simulink model "four_phase_iek_dynamic_load_refslew"  (R2024b)
settings: Solver=VariableStepAuto  StartTime=0.0  StopTime=2e-3  MaxStep=max_step_cont  RelTol=1e-3
undefined symbols (not defined in the file): Cout, DCR_L1, DCR_L2, DCR_L3, DCR_L4, ESR_C, IL_adc_counts_per_A, IL_pk_limit_adc_neg, IL_pk_limit_adc_pos, Iload_final, Iload_initial, Iqcot_enable, Kiqcot, L, Lambda1, Lambda2, Lambda3, Lambda4, Ri_area, t_load_step, Tblank, Tdead, Tiqcot_leak, Toff_min, Ton_cmd, Ton_iq_max, Ton_iq_min, Ton_trim1, Ton_trim2, Ton_trim3, Ton_trim4, Tslot, Tss, Varea_bias, Vcot_ramp_amp, Vcot_ramp_enable, Vhys, Vin, Vo_ref
libraries: simulink x29, spsCurrentMeasurementLib x8, spsMosfetLib x8, spsSeriesRLCBranchLib x5, spsVoltageMeasurementLib x5, spsDCVoltageSourceLib x4, spsControlledCurrentSourceLib x1, spsGroundLib x1, spspowerguiLib x1
settings Model: Creator=zengruize  LastModifiedBy=zengruize

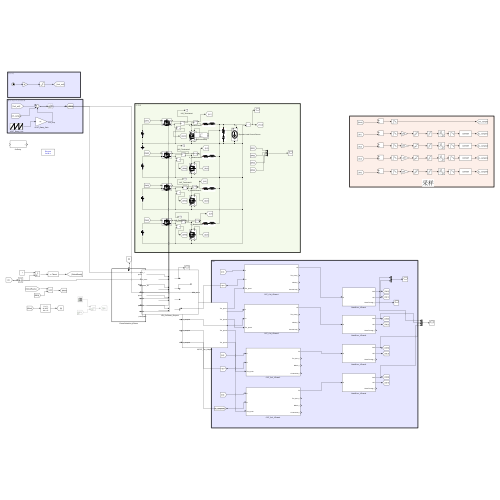
[thumbnail: Simulink's stored preview of the top-level diagram]
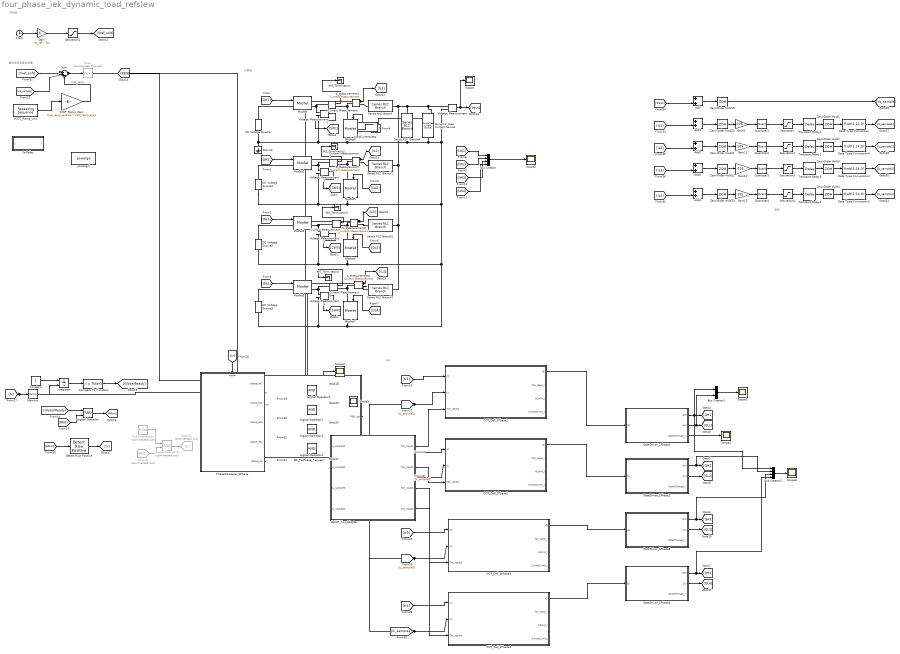
== system four_phase_iek_dynamic_load_refslew ==
  note: cot
  note: 输出电压误差比较器
  note: 功率级
  note: 软启动
  note: 采样
  Add{,1..4} (5 alike) : Sum
  Bus Creator : BusCreator  Inputs=4
  Bus Creator1 : BusCreator  Inputs=2
  Bus Creator2 : BusCreator  Inputs=4
  COT_Cell_1Phase1 : Subsystem
  COT_Cell_1Phase2 : Subsystem
  COT_Cell_1Phase3 : Subsystem
  COT_Cell_1Phase4 : Subsystem
  Clock : Clock
  Compare To Constant : simulink/Logic and Bit Operations/Compare To Constant  relop=>=  const=Tblank  OutDataTypeStr=boolean
  Constant : Constant
  Current Measurement{,1..3} (4 alike) : spsCurrentMeasurementLib/Current Measurement  PhasorSimulation=off  OutputType=Complex  PSBequivalent=0
  DC Voltage Source{,1..3} (4 alike) : spsDCVoltageSourceLib/DC Voltage Source  Amplitude=Vin  Measurements=None
  Data Type Conversion{,2..4} (4 alike) : DataTypeConversion  OutDataTypeStr=fixdt(1,14,0)  SaturateOnIntegerOverflow=off  RndMeth=Floor
  Detect Rise Positive : simulink/Logic and Bit Operations/Detect Rise Positive  vinit=0  OutDataTypeStr=boolean
  Dynamic Load Current Source : spsControlledCurrentSourceLib/Controlled Current Source  Initialize=on  Source_Type=DC  Amplitude=0  Phase=0  Frequency=0  Measurements=None
  From31 : From  Commented=on  GotoTag=REQ
  Gain : Gain  Gain=Vo_ref / Tss
  Gain11 : Gain  Gain=205
  Gain12 : Gain  Gain=-205
  Gain13 : Gain  Gain=205
  Gain9 : Gain  Gain=-205
  GateDriver_1Phase1 : Subsystem
  GateDriver_1Phase2 : Subsystem
  GateDriver_1Phase3 : Subsystem
  GateDriver_1Phase4 : Subsystem
  Goto26 : Goto  Commented=on  GotoTag=tr
  Ground : spsGroundLib/Ground  LConnTagsString=a
  IEK_PerPhase_Request : Subsystem
  IHS_Terminator{1..4} (4 alike) : Terminator
  IL_Measurement{1..4} (4 alike) : spsCurrentMeasurementLib/Current Measurement  PhasorSimulation=off  OutputType=Complex  PSBequivalent=0
  IQCOT_Ton_Adapter : Subsystem
  Integrator : Integrator  ExternalReset=rising
  LoadCurrentStep : Step  Time=t_load_step  Before=Iload_initial  After=Iload_final  SampleTime=0
  Logical Operator{,1..4} (5 alike) : Logic  AllPortsSameDT=off  OutDataTypeStr=boolean
  Logical Operator5 : Logic  Commented=on  AllPortsSameDT=off  OutDataTypeStr=boolean
  Memory : Memory
  Mosfet{,1..3} (4 alike) : spsMosfetLib/Mosfet  Ron=Ron_HS  Lon=0  Rd=Rd_body  Vfd=Vfd_body  IC=0  Rs=Rs_snubber  Cs=Cs_snubber  Measurements=on
  Mosfet{4..7} (4 alike) : spsMosfetLib/Mosfet  Ron=Ron_LS  Lon=0  Rd=Rd_body  Vfd=Vfd_body  IC=0  Rs=Rs_snubber  Cs=Cs_snubber  Measurements=on
  OnDelay : Subsystem
  PhaseScheduler_4Phase : Subsystem  TreatAsAtomicUnit=on
  Pulse Generator : DiscretePulseGenerator  Commented=on  PulseType=Time based  Period=Tblank  PulseWidth=5
  Quantizer{1..4} (4 alike) : Quantizer  QuantizationInterval=1
  Relay : Relay  Commented=through  OnSwitchValue=Vhys/2  OffSwitchValue=-Vhys/2
  Saturation{,1,3..4} (4 alike) : Saturate  UpperLimit=8191  LowerLimit=-8191
  Saturation2 : Saturate  UpperLimit=Vo_ref  LowerLimit=0
  Scope{,1..6} (7 alike) : Scope
  Series RLC Branch : spsSeriesRLCBranchLib/Series RLC Branch  LConnTagsString=__new0  RConnTagsString=__new0  BranchType=RL  Resistance=DCR_L1  Inductance=L  SetiL0=off  InitialCurrent=0  Capacitance=1e-6  Setx0=off  InitialVoltage=0  Measurements=None
  Series RLC Branch1 : spsSeriesRLCBranchLib/Series RLC Branch  LConnTagsString=__new0  RConnTagsString=__new0  BranchType=RL  Resistance=DCR_L2  Inductance=L  SetiL0=off  InitialCurrent=0  Capacitance=1e-6  Setx0=off  InitialVoltage=0  Measurements=None
  Series RLC Branch2 : spsSeriesRLCBranchLib/Series RLC Branch  LConnTagsString=__new0  RConnTagsString=__new0  BranchType=RL  Resistance=DCR_L3  Inductance=L  SetiL0=off  InitialCurrent=0  Capacitance=1e-6  Setx0=off  InitialVoltage=0  Measurements=None
  Series RLC Branch3 : spsSeriesRLCBranchLib/Series RLC Branch  LConnTagsString=__new0  RConnTagsString=__new0  BranchType=RL  Resistance=DCR_L4  Inductance=L  SetiL0=off  InitialCurrent=0  Capacitance=1e-6  Setx0=off  InitialVoltage=0  Measurements=None
  Series RLC Branch4 : spsSeriesRLCBranchLib/Series RLC Branch  LConnTagsString=__new0  RConnTagsString=__new0  BranchType=RC  Resistance=ESR_C  Inductance=1e-3  SetiL0=off  InitialCurrent=0  Capacitance=Cout  Setx0=on  InitialVoltage=Vo_ref  Measurements=None
  Sum : Sum  Inputs=|+--
  Transport Delay{1..4} (4 alike) : TransportDelay  DelayTime=5/25000000
  VCOT_Ramp_Gain : Gain  Gain=Vcot_ramp_enable * Vcot_ramp_amp
  VCOT_Ramp_Unit : simulink/Sources/Repeating Sequence  rep_seq_t=[0 Tslot]  rep_seq_y=[0 1]
  Voltage Measurement{,1..4} (5 alike) : spsVoltageMeasurementLib/Voltage Measurement  PhasorSimulation=off  OutputType=Complex  PSBequivalent=0
  Zero-Order Hold{1..4,19..23} (9 alike) : ZeroOrderHold  SampleTime=1/25000000
  powergui : spspowerguiLib/powergui  Priority=1  SimulationMode=Discrete  SampleTime=2e-9  frequency=60  Iterations=50  frequencyindice=0  Pbase=100e6  ErrMax=1e-4  UnitsV=kV  UnitsW=MW  buscounter=0  FunctionMessages=off  echomessages=off  EnableUseOfTLC=off  CurrentSourceSwitches=off  DisableSnubberDevices=off  DisableRonSwitches=off  DisableVfSwitches=off  DisplayEquations=off  AutomaticDiscreteSolvers=off  SolverType=Tustin/Backward Euler (TBE)  Interpol=off  ExternalGateDelay=off  methode=off  Ts=100  x0status=blocks  SPID=on  SwTol=0  HookPort=off  NonlinearTolerance=1e-4  nMaxIteration=100  ContinueOnMaxIteration=off  RestoreLinks=warning  ResistiveCurrentMeasurement=off  Frange=[0:2:500]  Ylog=off  Xlog=on  ShowGrid=off  save=off  variable=ZData  structure=0  ZoomFFT=off  StartTime=0.0  cycles=1  DisplayStyle=1  fundamental=60  FreqAxis=off  MaxFrequency=1000  frequencyindicesteady=1  RmsSteady=1  display=off
  wires:
  [QH1] -> Mosfet/1
  [QH4] -> Mosfet3/1
  [QH2] -> Mosfet1/1
  [QH3] -> Mosfet2/1
  [QL1] -> Mosfet4/1
  [QL2] -> Mosfet5/1
  [QL3] -> Mosfet6/1
  [QL4] -> Mosfet7/1
  Voltage Measurement2/1 -> [SW2]
  Voltage Measurement3/1 -> [SW3]
  Voltage Measurement1/1 -> [SW1]
  Voltage Measurement4/1 -> [SW4]
  GateDriver_1Phase1/1(QHi) -> Bus Creator1/1, [QH1], Bus Creator2/1
  GateDriver_1Phase2/1(QHi) -> Bus Creator2/2, [QH2]
  GateDriver_1Phase3/1(QHi) -> Bus Creator2/3, [QH3]
  GateDriver_1Phase4/1(QHi) -> Bus Creator2/4, [QH4]
  GateDriver_1Phase1/2(QLi) -> Bus Creator1/2, [QL1]
  GateDriver_1Phase2/2(QLi) -> [QL2]
  GateDriver_1Phase3/2(QLi) -> [QL3]
  GateDriver_1Phase4/2(QLi) -> [QL4]
  COT_Cell_1Phase1/1(Qi) -> GateDriver_1Phase1/1(Qi)
  COT_Cell_1Phase2/1(Qi) -> GateDriver_1Phase2/1(Qi)
  COT_Cell_1Phase3/1(Qi) -> GateDriver_1Phase3/1(Qi)
  COT_Cell_1Phase4/1(Qi) -> GateDriver_1Phase4/1(Qi)
  GateDriver_1Phase1/3(ShootThrough_i) -> Scope1/1
  Bus Creator/1 -> Scope2/1
  [SW1] -> Bus Creator/1
  [SW2] -> Bus Creator/2
  [SW3] -> Bus Creator/3
  [SW4] -> Bus Creator/4
  Bus Creator1/1 -> Scope3/1
  Saturation2/1 -> [Vref_soft]
  Gain/1 -> Saturation2/1
  Clock/1 -> Gain/1
  Voltage Measurement/1 -> Scope/1, [Vout]
  [Vref_soft] -> Sum/1
  [Vo_sample] -> Sum/2
  Sum/1 -> Relay/1, IEK_PerPhase_Request/1(e_v)
  Constant/1 -> Integrator/1
  Integrator/1 -> Compare To Constant/1
  Compare To Constant/1 -> [GlobalReady]
  [GlobalReady] -> Logical Operator/1
  [REQ] -> Logical Operator/2
  Logical Operator/1 -> [Allow]
  [Allow] -> Detect Rise Positive/1
  Detect Rise Positive/1 -> [tr]
  [tr] -> PhaseScheduler_4Phase/Trigger
  PhaseScheduler_4Phase/1(phase_en1) -> Logical Operator1/1
  [tr] -> Logical Operator1/2
  PhaseScheduler_4Phase/2(phase_en2) -> Logical Operator2/1
  [tr] -> Logical Operator2/2
  PhaseScheduler_4Phase/3(phase_en3) -> Logical Operator3/1
  [tr] -> Logical Operator3/2
  PhaseScheduler_4Phase/4(phase_en4) -> Logical Operator4/1
  [tr] -> Logical Operator4/2
  Logical Operator1/1 -> Scope4/1, [tr1]
  Logical Operator2/1 -> Scope5/1, [tr2]
  Logical Operator3/1 -> [tr3]
  Logical Operator4/1 -> [tr4]
  [tr1] -> COT_Cell_1Phase1/1(tri)
  [tr2] -> COT_Cell_1Phase2/1(tri)
  [tr3] -> COT_Cell_1Phase3/1(tri)
  [tr4] -> COT_Cell_1Phase4/1(tri)
  [IL_sample1] -> COT_Cell_1Phase1/2(ILi), IQCOT_Ton_Adapter/1(IL_sample1)
  [IL_sample2] -> COT_Cell_1Phase2/2(ILi), IQCOT_Ton_Adapter/2(IL_sample2)
  [IL_sample3] -> COT_Cell_1Phase3/2(ILi), IQCOT_Ton_Adapter/3(IL_sample3)
  [IL_sample4] -> COT_Cell_1Phase4/2(ILi), IQCOT_Ton_Adapter/4(IL_sample4)
  [tr] -> Memory/1, IEK_PerPhase_Request/2(tr_reset)
  Memory/1 -> Integrator/2
  Logical Operator5/1 -> Goto26/1
  Pulse Generator/1 -> Logical Operator5/1
  From31/1 -> Logical Operator5/2
  Bus Creator2/1 -> Scope6/1
  IL_Measurement1/1 -> [IL1], IEK_PerPhase_Request/4(IL1)
  IL_Measurement2/1 -> [IL2], IEK_PerPhase_Request/5(IL2)
  IL_Measurement3/1 -> [IL3], IEK_PerPhase_Request/6(IL3)
  IL_Measurement4/1 -> [IL4], IEK_PerPhase_Request/7(IL4)
  Current Measurement/1 -> IHS_Terminator1/1
  Current Measurement1/1 -> IHS_Terminator2/1
  Current Measurement2/1 -> IHS_Terminator3/1
  Current Measurement3/1 -> IHS_Terminator4/1
  Zero-Order Hold23/1 -> Gain13/1
  Zero-Order Hold20/1 -> Gain9/1
  Zero-Order Hold3/1 -> Data Type Conversion3/1
  Zero-Order Hold4/1 -> Data Type Conversion2/1
  Saturation4/1 -> Transport Delay4/1
  Zero-Order Hold1/1 -> Data Type Conversion/1
  [IL3] -> Add3/2
  Add3/1 -> Zero-Order Hold22/1
  Quantizer1/1 -> Saturation/1
  Quantizer4/1 -> Saturation4/1
  Gain12/1 -> Quantizer3/1
  [IL4] -> Add4/2
  Add/1 -> Zero-Order Hold19/1
  Data Type Conversion/1 -> [IL_sample1]
  Data Type Conversion2/1 -> [IL_sample4]
  Add4/1 -> Zero-Order Hold23/1
  Transport Delay3/1 -> Zero-Order Hold3/1
  Saturation3/1 -> Transport Delay3/1
  Add1/1 -> Zero-Order Hold20/1
  [IL1] -> Add1/2
  Transport Delay4/1 -> Zero-Order Hold4/1
  Zero-Order Hold21/1 -> Gain11/1
  Data Type Conversion3/1 -> [IL_sample3]
  Gain9/1 -> Quantizer1/1
  Gain11/1 -> Quantizer2/1
  Saturation/1 -> Transport Delay1/1
  [IL2] -> Add2/2
  Transport Delay2/1 -> Zero-Order Hold2/1
  Zero-Order Hold19/1 -> [Vo_sample]
  Gain13/1 -> Quantizer4/1
  Quantizer3/1 -> Saturation3/1
  Data Type Conversion4/1 -> [IL_sample2]
  Zero-Order Hold2/1 -> Data Type Conversion4/1
  Add2/1 -> Zero-Order Hold21/1
  Transport Delay1/1 -> Zero-Order Hold1/1
  [Vout] -> Add/2
  Saturation1/1 -> Transport Delay2/1
  Zero-Order Hold22/1 -> Gain12/1
  Quantizer2/1 -> Saturation1/1
  VCOT_Ramp_Unit/1 -> VCOT_Ramp_Gain/1
  VCOT_Ramp_Gain/1 -> Sum/3  "Vcot_ramp"
  IQCOT_Ton_Adapter/1(Ton_iqcot1) -> COT_Cell_1Phase1/3(Ton_iqcot1)
  IQCOT_Ton_Adapter/2(Ton_iqcot2) -> COT_Cell_1Phase2/3(Ton_iqcot2)
  IQCOT_Ton_Adapter/3(Ton_iqcot3) -> COT_Cell_1Phase3/3(Ton_iqcot3)
  IQCOT_Ton_Adapter/4(Ton_iqcot4) -> COT_Cell_1Phase4/3(Ton_iqcot4)
  PhaseScheduler_4Phase/5(phase_idx) -> IEK_PerPhase_Request/3(phase_idx)
  IEK_PerPhase_Request/1(REQ_iek) -> [REQ]
  LoadCurrentStep/1 -> Dynamic Load Current Source/1
  connections:
  DC Voltage Source/LConn1 -- Voltage Measurement1/LConn2 -- Mosfet7/RConn1 -- Voltage Measurement4/LConn2 -- DC Voltage Source3/LConn1 -- Mosfet6/RConn1 -- Voltage Measurement3/LConn2 -- DC Voltage Source2/LConn1 -- DC Voltage Source1/LConn1 -- Voltage Measurement2/LConn2 -- Mosfet5/RConn1 -- Voltage Measurement/LConn2 -- Dynamic Load Current Source/RConn1 -- Series RLC Branch4/RConn1 -- Mosfet4/RConn1 -- Ground/LConn1
  Mosfet/LConn1 -- DC Voltage Source/RConn1
  DC Voltage Source1/RConn1 -- Mosfet1/LConn1
  Mosfet1/RConn1 -- Current Measurement1/LConn1 -- Voltage Measurement2/LConn1
  DC Voltage Source2/RConn1 -- Mosfet2/LConn1
  Mosfet2/RConn1 -- Current Measurement2/LConn1 -- Voltage Measurement3/LConn1
  DC Voltage Source3/RConn1 -- Mosfet3/LConn1
  Series RLC Branch/RConn1 -- Series RLC Branch3/RConn1 -- Series RLC Branch2/RConn1 -- Series RLC Branch1/RConn1 -- Voltage Measurement/LConn1 -- Dynamic Load Current Source/LConn1 -- Series RLC Branch4/LConn1
  Mosfet/RConn1 -- Current Measurement/LConn1 -- Voltage Measurement1/LConn1
  Mosfet3/RConn1 -- Current Measurement3/LConn1 -- Voltage Measurement4/LConn1
  Current Measurement/RConn1 -- Mosfet4/LConn1 -- IL_Measurement1/LConn1
  IL_Measurement1/RConn1 -- Series RLC Branch/LConn1
  Current Measurement1/RConn1 -- Mosfet5/LConn1 -- IL_Measurement2/LConn1
  IL_Measurement2/RConn1 -- Series RLC Branch1/LConn1
  Mosfet6/LConn1 -- Current Measurement2/RConn1 -- IL_Measurement3/LConn1
  IL_Measurement3/RConn1 -- Series RLC Branch2/LConn1
  Current Measurement3/RConn1 -- Mosfet7/LConn1 -- IL_Measurement4/LConn1
  IL_Measurement4/RConn1 -- Series RLC Branch3/LConn1

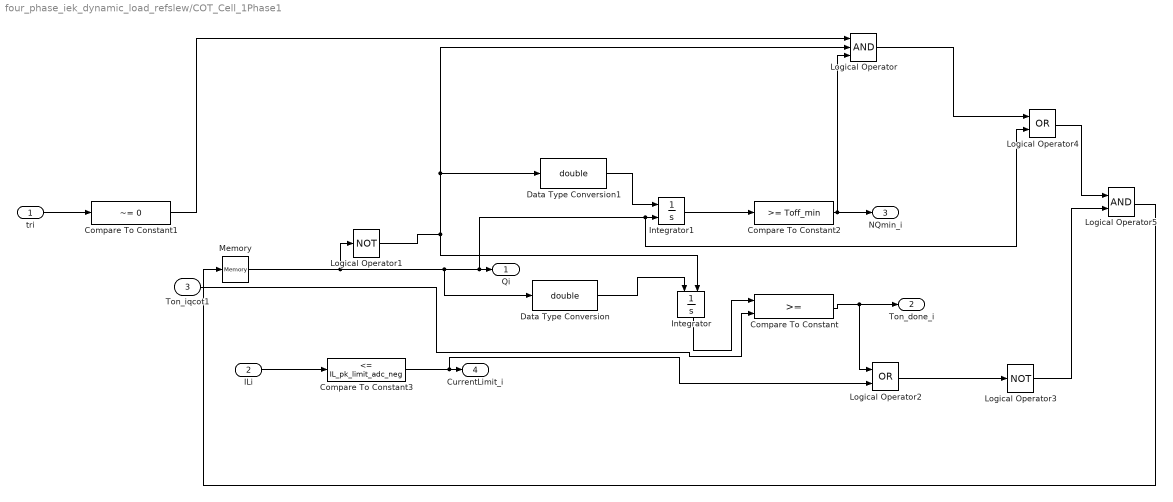
== system four_phase_iek_dynamic_load_refslew/COT_Cell_1Phase1 ==
  tri : Inport
  ILi : Inport  Port=2
  Ton_iqcot1 : Inport  Port=3
  Compare To Constant : RelationalOperator  OutDataTypeStr=boolean  RndMeth=Simplest  InputSameDT=off
  Compare To Constant1 : simulink/Logic and Bit Operations/Compare To Constant  relop=~=  const=0  OutDataTypeStr=boolean
  Compare To Constant2 : simulink/Logic and Bit Operations/Compare To Constant  relop=>=  const=Toff_min  OutDataTypeStr=boolean
  Compare To Constant3 : simulink/Logic and Bit Operations/Compare To Constant  relop=<=  const=IL_pk_limit_adc_neg  OutDataTypeStr=boolean
  Data Type Conversion : DataTypeConversion  OutDataTypeStr=double  SaturateOnIntegerOverflow=off  RndMeth=Floor
  Data Type Conversion1 : DataTypeConversion  OutDataTypeStr=double  SaturateOnIntegerOverflow=off  RndMeth=Floor
  Integrator : Integrator  ExternalReset=level
  Integrator1 : Integrator  ExternalReset=level  InitialCondition=Toff_min
  Logical Operator : Logic  Inputs=3  AllPortsSameDT=off  OutDataTypeStr=boolean
  Logical Operator1 : Logic  Operator=NOT  AllPortsSameDT=off  OutDataTypeStr=boolean
  Logical Operator2 : Logic  Operator=OR  AllPortsSameDT=off  OutDataTypeStr=boolean
  Logical Operator3 : Logic  Operator=NOT  Inputs=3  AllPortsSameDT=off  OutDataTypeStr=boolean
  Logical Operator4 : Logic  Operator=OR  AllPortsSameDT=off  OutDataTypeStr=boolean
  Logical Operator5 : Logic  AllPortsSameDT=off  OutDataTypeStr=boolean
  Memory : Memory
  Qi : Outport
  Ton_done_i : Outport  Port=2
  NQmin_i : Outport  Port=3
  CurrentLimit_i : Outport  Port=4
  wires:
  Compare To Constant/1 -> Logical Operator2/1, Ton_done_i/1
  tri/1 -> Compare To Constant1/1
  Compare To Constant1/1 -> Logical Operator/1
  Memory/1 -> Logical Operator1/1, Data Type Conversion/1, Logical Operator4/2, Integrator1/2, Qi/1
  Logical Operator1/1 -> Data Type Conversion1/1, Logical Operator/2, Integrator/2
  Data Type Conversion/1 -> Integrator/1
  Integrator/1 -> Compare To Constant/1
  Data Type Conversion1/1 -> Integrator1/1
  Integrator1/1 -> Compare To Constant2/1
  Compare To Constant2/1 -> Logical Operator/3, NQmin_i/1
  ILi/1 -> Compare To Constant3/1
  Compare To Constant3/1 -> Logical Operator2/2, CurrentLimit_i/1
  Logical Operator2/1 -> Logical Operator3/1
  Logical Operator/1 -> Logical Operator4/1
  Logical Operator4/1 -> Logical Operator5/1
  Logical Operator3/1 -> Logical Operator5/2
  Logical Operator5/1 -> Memory/1
  Ton_iqcot1/1 -> Compare To Constant/2

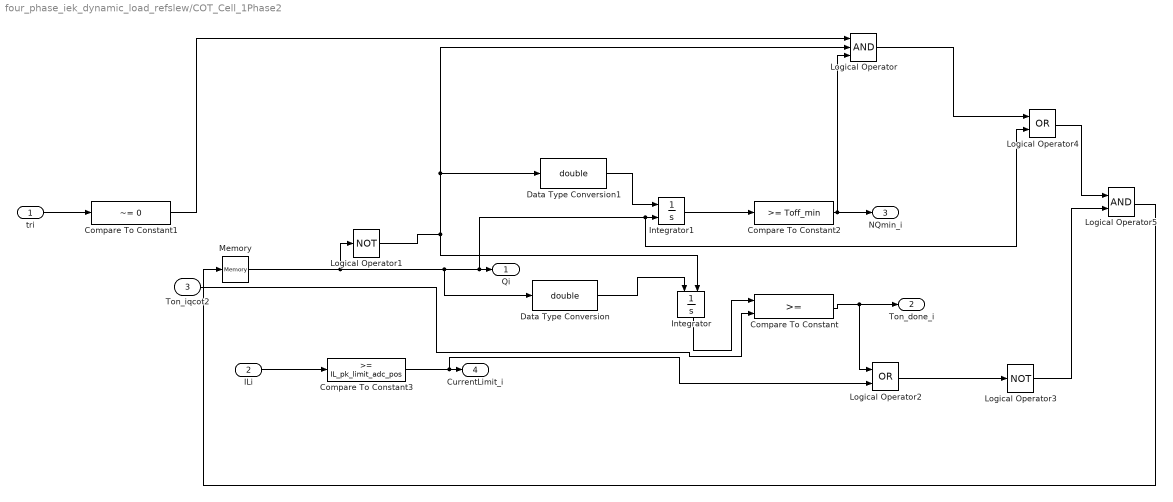
== system four_phase_iek_dynamic_load_refslew/COT_Cell_1Phase2 ==
  tri : Inport
  ILi : Inport  Port=2
  Ton_iqcot2 : Inport  Port=3
  Compare To Constant : RelationalOperator  OutDataTypeStr=boolean  RndMeth=Simplest  InputSameDT=off
  Compare To Constant1 : simulink/Logic and Bit Operations/Compare To Constant  relop=~=  const=0  OutDataTypeStr=boolean
  Compare To Constant2 : simulink/Logic and Bit Operations/Compare To Constant  relop=>=  const=Toff_min  OutDataTypeStr=boolean
  Compare To Constant3 : simulink/Logic and Bit Operations/Compare To Constant  relop=>=  const=IL_pk_limit_adc_pos  OutDataTypeStr=boolean
  Data Type Conversion : DataTypeConversion  OutDataTypeStr=double  SaturateOnIntegerOverflow=off  RndMeth=Floor
  Data Type Conversion1 : DataTypeConversion  OutDataTypeStr=double  SaturateOnIntegerOverflow=off  RndMeth=Floor
  Integrator : Integrator  ExternalReset=level
  Integrator1 : Integrator  ExternalReset=level  InitialCondition=Toff_min
  Logical Operator : Logic  Inputs=3  AllPortsSameDT=off  OutDataTypeStr=boolean
  Logical Operator1 : Logic  Operator=NOT  AllPortsSameDT=off  OutDataTypeStr=boolean
  Logical Operator2 : Logic  Operator=OR  AllPortsSameDT=off  OutDataTypeStr=boolean
  Logical Operator3 : Logic  Operator=NOT  Inputs=3  AllPortsSameDT=off  OutDataTypeStr=boolean
  Logical Operator4 : Logic  Operator=OR  AllPortsSameDT=off  OutDataTypeStr=boolean
  Logical Operator5 : Logic  AllPortsSameDT=off  OutDataTypeStr=boolean
  Memory : Memory
  Qi : Outport
  Ton_done_i : Outport  Port=2
  NQmin_i : Outport  Port=3
  CurrentLimit_i : Outport  Port=4
  wires:
  Compare To Constant/1 -> Logical Operator2/1, Ton_done_i/1
  tri/1 -> Compare To Constant1/1
  Compare To Constant1/1 -> Logical Operator/1
  Memory/1 -> Logical Operator1/1, Data Type Conversion/1, Logical Operator4/2, Integrator1/2, Qi/1
  Logical Operator1/1 -> Data Type Conversion1/1, Logical Operator/2, Integrator/2
  Data Type Conversion/1 -> Integrator/1
  Integrator/1 -> Compare To Constant/1
  Data Type Conversion1/1 -> Integrator1/1
  Integrator1/1 -> Compare To Constant2/1
  Compare To Constant2/1 -> Logical Operator/3, NQmin_i/1
  ILi/1 -> Compare To Constant3/1
  Compare To Constant3/1 -> Logical Operator2/2, CurrentLimit_i/1
  Logical Operator2/1 -> Logical Operator3/1
  Logical Operator/1 -> Logical Operator4/1
  Logical Operator4/1 -> Logical Operator5/1
  Logical Operator3/1 -> Logical Operator5/2
  Logical Operator5/1 -> Memory/1
  Ton_iqcot2/1 -> Compare To Constant/2

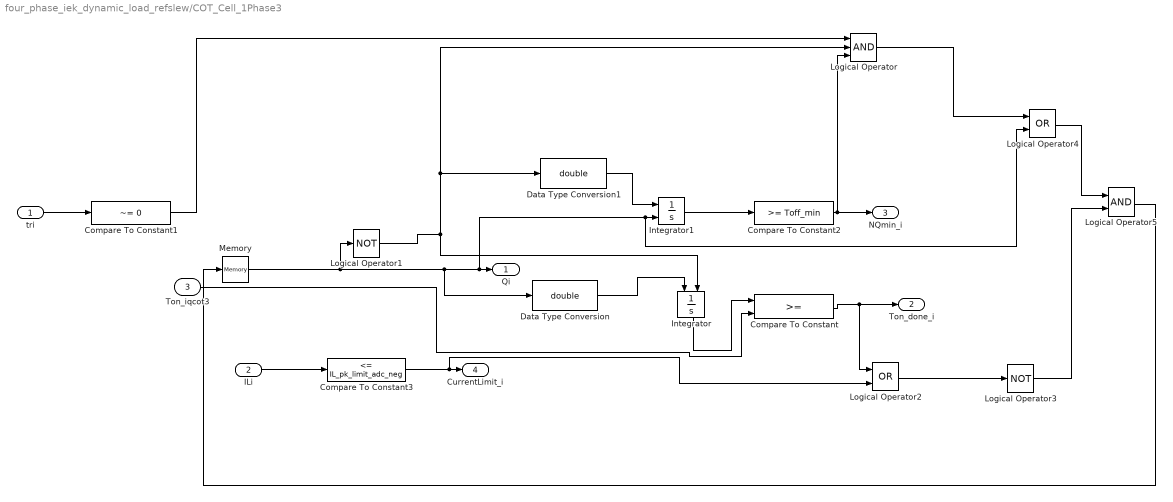
== system four_phase_iek_dynamic_load_refslew/COT_Cell_1Phase3 ==
  tri : Inport
  ILi : Inport  Port=2
  Ton_iqcot3 : Inport  Port=3
  Compare To Constant : RelationalOperator  OutDataTypeStr=boolean  RndMeth=Simplest  InputSameDT=off
  Compare To Constant1 : simulink/Logic and Bit Operations/Compare To Constant  relop=~=  const=0  OutDataTypeStr=boolean
  Compare To Constant2 : simulink/Logic and Bit Operations/Compare To Constant  relop=>=  const=Toff_min  OutDataTypeStr=boolean
  Compare To Constant3 : simulink/Logic and Bit Operations/Compare To Constant  relop=<=  const=IL_pk_limit_adc_neg  OutDataTypeStr=boolean
  Data Type Conversion : DataTypeConversion  OutDataTypeStr=double  SaturateOnIntegerOverflow=off  RndMeth=Floor
  Data Type Conversion1 : DataTypeConversion  OutDataTypeStr=double  SaturateOnIntegerOverflow=off  RndMeth=Floor
  Integrator : Integrator  ExternalReset=level
  Integrator1 : Integrator  ExternalReset=level  InitialCondition=Toff_min
  Logical Operator : Logic  Inputs=3  AllPortsSameDT=off  OutDataTypeStr=boolean
  Logical Operator1 : Logic  Operator=NOT  AllPortsSameDT=off  OutDataTypeStr=boolean
  Logical Operator2 : Logic  Operator=OR  AllPortsSameDT=off  OutDataTypeStr=boolean
  Logical Operator3 : Logic  Operator=NOT  Inputs=3  AllPortsSameDT=off  OutDataTypeStr=boolean
  Logical Operator4 : Logic  Operator=OR  AllPortsSameDT=off  OutDataTypeStr=boolean
  Logical Operator5 : Logic  AllPortsSameDT=off  OutDataTypeStr=boolean
  Memory : Memory
  Qi : Outport
  Ton_done_i : Outport  Port=2
  NQmin_i : Outport  Port=3
  CurrentLimit_i : Outport  Port=4
  wires:
  Compare To Constant/1 -> Logical Operator2/1, Ton_done_i/1
  tri/1 -> Compare To Constant1/1
  Compare To Constant1/1 -> Logical Operator/1
  Memory/1 -> Logical Operator1/1, Data Type Conversion/1, Logical Operator4/2, Integrator1/2, Qi/1
  Logical Operator1/1 -> Data Type Conversion1/1, Logical Operator/2, Integrator/2
  Data Type Conversion/1 -> Integrator/1
  Integrator/1 -> Compare To Constant/1
  Data Type Conversion1/1 -> Integrator1/1
  Integrator1/1 -> Compare To Constant2/1
  Compare To Constant2/1 -> Logical Operator/3, NQmin_i/1
  ILi/1 -> Compare To Constant3/1
  Compare To Constant3/1 -> Logical Operator2/2, CurrentLimit_i/1
  Logical Operator2/1 -> Logical Operator3/1
  Logical Operator/1 -> Logical Operator4/1
  Logical Operator4/1 -> Logical Operator5/1
  Logical Operator3/1 -> Logical Operator5/2
  Logical Operator5/1 -> Memory/1
  Ton_iqcot3/1 -> Compare To Constant/2

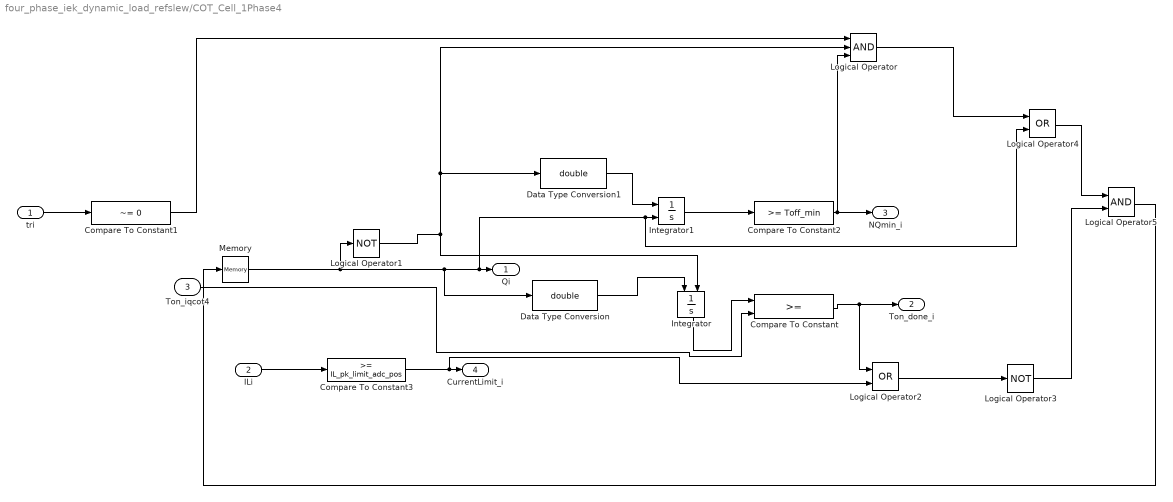
== system four_phase_iek_dynamic_load_refslew/COT_Cell_1Phase4 ==
  tri : Inport
  ILi : Inport  Port=2
  Ton_iqcot4 : Inport  Port=3
  Compare To Constant : RelationalOperator  OutDataTypeStr=boolean  RndMeth=Simplest  InputSameDT=off
  Compare To Constant1 : simulink/Logic and Bit Operations/Compare To Constant  relop=~=  const=0  OutDataTypeStr=boolean
  Compare To Constant2 : simulink/Logic and Bit Operations/Compare To Constant  relop=>=  const=Toff_min  OutDataTypeStr=boolean
  Compare To Constant3 : simulink/Logic and Bit Operations/Compare To Constant  relop=>=  const=IL_pk_limit_adc_pos  OutDataTypeStr=boolean
  Data Type Conversion : DataTypeConversion  OutDataTypeStr=double  SaturateOnIntegerOverflow=off  RndMeth=Floor
  Data Type Conversion1 : DataTypeConversion  OutDataTypeStr=double  SaturateOnIntegerOverflow=off  RndMeth=Floor
  Integrator : Integrator  ExternalReset=level
  Integrator1 : Integrator  ExternalReset=level  InitialCondition=Toff_min
  Logical Operator : Logic  Inputs=3  AllPortsSameDT=off  OutDataTypeStr=boolean
  Logical Operator1 : Logic  Operator=NOT  AllPortsSameDT=off  OutDataTypeStr=boolean
  Logical Operator2 : Logic  Operator=OR  AllPortsSameDT=off  OutDataTypeStr=boolean
  Logical Operator3 : Logic  Operator=NOT  Inputs=3  AllPortsSameDT=off  OutDataTypeStr=boolean
  Logical Operator4 : Logic  Operator=OR  AllPortsSameDT=off  OutDataTypeStr=boolean
  Logical Operator5 : Logic  AllPortsSameDT=off  OutDataTypeStr=boolean
  Memory : Memory
  Qi : Outport
  Ton_done_i : Outport  Port=2
  NQmin_i : Outport  Port=3
  CurrentLimit_i : Outport  Port=4
  wires:
  Compare To Constant/1 -> Logical Operator2/1, Ton_done_i/1
  tri/1 -> Compare To Constant1/1
  Compare To Constant1/1 -> Logical Operator/1
  Memory/1 -> Logical Operator1/1, Data Type Conversion/1, Logical Operator4/2, Integrator1/2, Qi/1
  Logical Operator1/1 -> Data Type Conversion1/1, Logical Operator/2, Integrator/2
  Data Type Conversion/1 -> Integrator/1
  Integrator/1 -> Compare To Constant/1
  Data Type Conversion1/1 -> Integrator1/1
  Integrator1/1 -> Compare To Constant2/1
  Compare To Constant2/1 -> Logical Operator/3, NQmin_i/1
  ILi/1 -> Compare To Constant3/1
  Compare To Constant3/1 -> Logical Operator2/2, CurrentLimit_i/1
  Logical Operator2/1 -> Logical Operator3/1
  Logical Operator/1 -> Logical Operator4/1
  Logical Operator4/1 -> Logical Operator5/1
  Logical Operator3/1 -> Logical Operator5/2
  Logical Operator5/1 -> Memory/1
  Ton_iqcot4/1 -> Compare To Constant/2

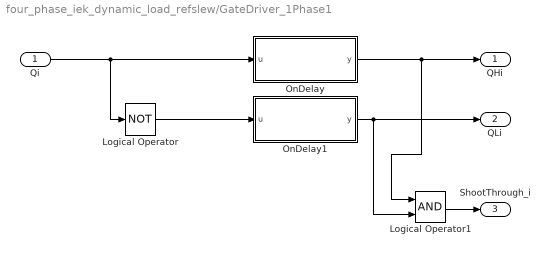
== system four_phase_iek_dynamic_load_refslew/GateDriver_1Phase1 ==
  Qi : Inport
  Logical Operator : Logic  Operator=NOT  AllPortsSameDT=off  OutDataTypeStr=boolean
  Logical Operator1 : Logic  AllPortsSameDT=off  OutDataTypeStr=boolean
  OnDelay : Subsystem
  OnDelay1 : Subsystem
  QHi : Outport
  QLi : Outport  Port=2
  ShootThrough_i : Outport  Port=3
  wires:
  Qi/1 -> Logical Operator/1, OnDelay/1(u)
  OnDelay/1(y) -> Logical Operator1/1, QHi/1
  Logical Operator/1 -> OnDelay1/1(u)
  OnDelay1/1(y) -> QLi/1, Logical Operator1/2
  Logical Operator1/1 -> ShootThrough_i/1

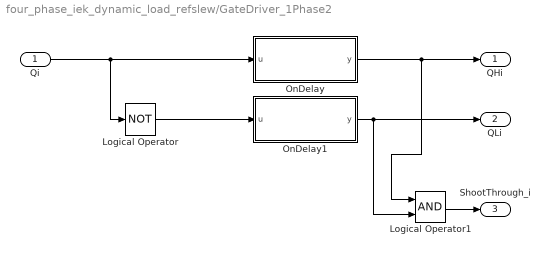
== system four_phase_iek_dynamic_load_refslew/GateDriver_1Phase2 ==
  Qi : Inport
  Logical Operator : Logic  Operator=NOT  AllPortsSameDT=off  OutDataTypeStr=boolean
  Logical Operator1 : Logic  AllPortsSameDT=off  OutDataTypeStr=boolean
  OnDelay : Subsystem
  OnDelay1 : Subsystem
  QHi : Outport
  QLi : Outport  Port=2
  ShootThrough_i : Outport  Port=3
  wires:
  Qi/1 -> Logical Operator/1, OnDelay/1(u)
  OnDelay/1(y) -> Logical Operator1/1, QHi/1
  Logical Operator/1 -> OnDelay1/1(u)
  OnDelay1/1(y) -> QLi/1, Logical Operator1/2
  Logical Operator1/1 -> ShootThrough_i/1

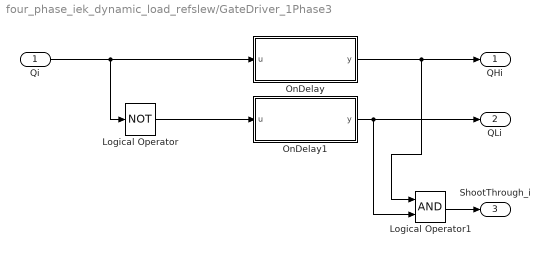
== system four_phase_iek_dynamic_load_refslew/GateDriver_1Phase3 ==
  Qi : Inport
  Logical Operator : Logic  Operator=NOT  AllPortsSameDT=off  OutDataTypeStr=boolean
  Logical Operator1 : Logic  AllPortsSameDT=off  OutDataTypeStr=boolean
  OnDelay : Subsystem
  OnDelay1 : Subsystem
  QHi : Outport
  QLi : Outport  Port=2
  ShootThrough_i : Outport  Port=3
  wires:
  Qi/1 -> Logical Operator/1, OnDelay/1(u)
  OnDelay/1(y) -> Logical Operator1/1, QHi/1
  Logical Operator/1 -> OnDelay1/1(u)
  OnDelay1/1(y) -> QLi/1, Logical Operator1/2
  Logical Operator1/1 -> ShootThrough_i/1

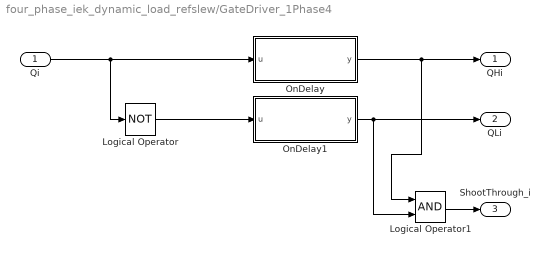
== system four_phase_iek_dynamic_load_refslew/GateDriver_1Phase4 ==
  Qi : Inport
  Logical Operator : Logic  Operator=NOT  AllPortsSameDT=off  OutDataTypeStr=boolean
  Logical Operator1 : Logic  AllPortsSameDT=off  OutDataTypeStr=boolean
  OnDelay : Subsystem
  OnDelay1 : Subsystem
  QHi : Outport
  QLi : Outport  Port=2
  ShootThrough_i : Outport  Port=3
  wires:
  Qi/1 -> Logical Operator/1, OnDelay/1(u)
  OnDelay/1(y) -> Logical Operator1/1, QHi/1
  Logical Operator/1 -> OnDelay1/1(u)
  OnDelay1/1(y) -> QLi/1, Logical Operator1/2
  Logical Operator1/1 -> ShootThrough_i/1

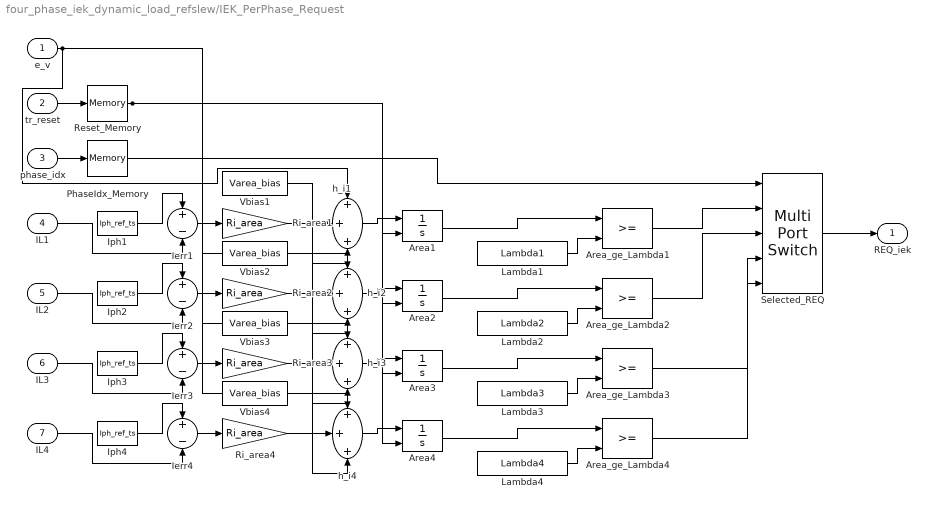
== system four_phase_iek_dynamic_load_refslew/IEK_PerPhase_Request ==
  e_v : Inport
  tr_reset : Inport  Port=2
  phase_idx : Inport  Port=3
  IL1 : Inport  Port=4
  IL2 : Inport  Port=5
  IL3 : Inport  Port=6
  IL4 : Inport  Port=7
  Area{1..4} (4 alike) : Integrator  ExternalReset=rising
  Area_ge_Lambda{1..4} (4 alike) : RelationalOperator  OutDataTypeStr=boolean  RndMeth=Simplest  InputSameDT=off
  Ierr{1..4} (4 alike) : Sum  Inputs=+-
  Iph{1..4} (4 alike) : FromWorkspace  VariableName=Iph_ref_ts  OutputAfterFinalValue=Holding final value
  Lambda1 : Constant  Value=Lambda1
  Lambda2 : Constant  Value=Lambda2
  Lambda3 : Constant  Value=Lambda3
  Lambda4 : Constant  Value=Lambda4
  PhaseIdx_Memory : Memory
  Reset_Memory : Memory
  Ri_area{1..4} (4 alike) : Gain  Gain=Ri_area
  Selected_REQ : MultiPortSwitch  DataPortOrder=Zero-based contiguous  Inputs=4  DiagnosticForDefault=None  zeroidx=on  SaturateOnIntegerOverflow=off  InputSameDT=off
  Vbias{1..4} (4 alike) : Constant  Value=Varea_bias
  h_i{1..4} (4 alike) : Sum  Inputs=+++
  REQ_iek : Outport
  wires:
  ? -> ?
  tr_reset/1 -> Reset_Memory/1
  phase_idx/1 -> PhaseIdx_Memory/1
  PhaseIdx_Memory/1 -> Selected_REQ/1
  Selected_REQ/1 -> REQ_iek/1
  IL1/1 -> Ierr1/2
  Ierr1/1 -> Ri_area1/1
  e_v/1 -> h_i1/1, h_i2/1, h_i3/1, h_i4/1
  Ri_area1/1 -> h_i1/2
  Vbias1/1 -> h_i1/3
  h_i1/1 -> Area1/1
  Reset_Memory/1 -> Area1/2, Area2/2, Area3/2, Area4/2
  Area1/1 -> Area_ge_Lambda1/1
  Lambda1/1 -> Area_ge_Lambda1/2
  Area_ge_Lambda1/1 -> Selected_REQ/2
  IL2/1 -> Ierr2/2
  Ierr2/1 -> Ri_area2/1
  Ri_area2/1 -> h_i2/2
  Vbias2/1 -> h_i2/3
  h_i2/1 -> Area2/1
  Area2/1 -> Area_ge_Lambda2/1
  Lambda2/1 -> Area_ge_Lambda2/2
  Area_ge_Lambda2/1 -> Selected_REQ/3
  IL3/1 -> Ierr3/2
  Ierr3/1 -> Ri_area3/1
  Ri_area3/1 -> h_i3/2
  Vbias3/1 -> h_i3/3
  h_i3/1 -> Area3/1
  Area3/1 -> Area_ge_Lambda3/1
  Lambda3/1 -> Area_ge_Lambda3/2
  Area_ge_Lambda3/1 -> Selected_REQ/4
  IL4/1 -> Ierr4/2
  Ierr4/1 -> Ri_area4/1
  Ri_area4/1 -> h_i4/2
  Vbias4/1 -> h_i4/3
  h_i4/1 -> Area4/1
  Area4/1 -> Area_ge_Lambda4/1
  Lambda4/1 -> Area_ge_Lambda4/2
  Area_ge_Lambda4/1 -> Selected_REQ/5
  Iph1/1 -> Ierr1/1
  Iph2/1 -> Ierr2/1
  Iph3/1 -> Ierr3/1
  Iph4/1 -> Ierr4/1

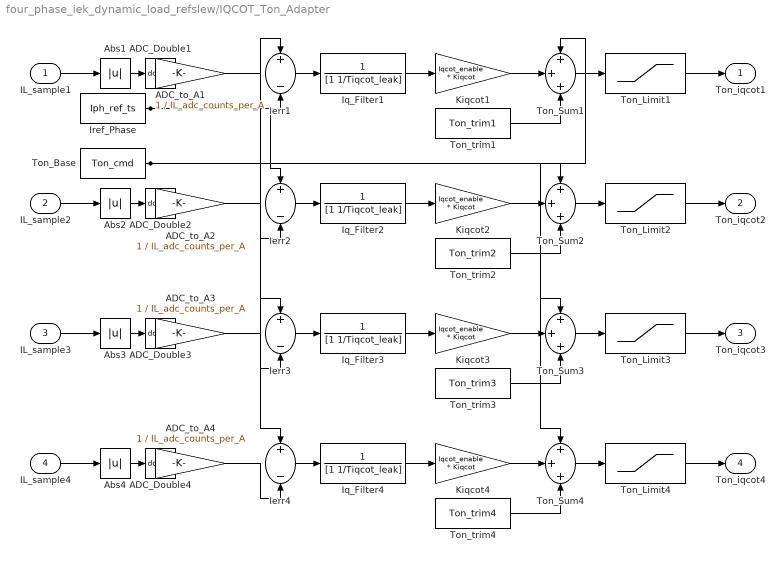
== system four_phase_iek_dynamic_load_refslew/IQCOT_Ton_Adapter ==
  IL_sample1 : Inport
  IL_sample2 : Inport  Port=2
  IL_sample3 : Inport  Port=3
  IL_sample4 : Inport  Port=4
  ADC_Double{1..4} (4 alike) : DataTypeConversion  OutDataTypeStr=double  SaturateOnIntegerOverflow=off  RndMeth=Floor
  ADC_to_A{1..4} (4 alike) : Gain  Gain=1 / IL_adc_counts_per_A  OutDataTypeStr=double
  Abs{1..4} (4 alike) : Abs  SaturateOnIntegerOverflow=off
  Ierr{1..4} (4 alike) : Sum  Inputs=+-
  Iq_Filter{1..4} (4 alike) : TransferFcn  Numerator=1  Denominator=[1 1/Tiqcot_leak]
  Iref_Phase : FromWorkspace  VariableName=Iph_ref_ts  OutputAfterFinalValue=Holding final value
  Kiqcot{1..4} (4 alike) : Gain  Gain=Iqcot_enable * Kiqcot
  Ton_Base : Constant  Value=Ton_cmd
  Ton_Limit{1..4} (4 alike) : Saturate  UpperLimit=Ton_iq_max  LowerLimit=Ton_iq_min
  Ton_Sum{1..4} (4 alike) : Sum  Inputs=+++
  Ton_trim1 : Constant  Value=Ton_trim1
  Ton_trim2 : Constant  Value=Ton_trim2
  Ton_trim3 : Constant  Value=Ton_trim3
  Ton_trim4 : Constant  Value=Ton_trim4
  Ton_iqcot1 : Outport
  Ton_iqcot2 : Outport  Port=2
  Ton_iqcot3 : Outport  Port=3
  Ton_iqcot4 : Outport  Port=4
  wires:
  ? -> ?
  IL_sample1/1 -> Abs1/1
  Abs1/1 -> ADC_Double1/1
  ADC_to_A1/1 -> Ierr1/2
  Ierr1/1 -> Iq_Filter1/1
  Iq_Filter1/1 -> Kiqcot1/1
  Kiqcot1/1 -> Ton_Sum1/2
  Ton_Base/1 -> Ton_Sum1/1, Ton_Sum2/1, Ton_Sum3/1, Ton_Sum4/1
  Ton_Sum1/1 -> Ton_Limit1/1
  Ton_Limit1/1 -> Ton_iqcot1/1
  IL_sample2/1 -> Abs2/1
  Abs2/1 -> ADC_Double2/1
  ADC_to_A2/1 -> Ierr2/2
  Ierr2/1 -> Iq_Filter2/1
  Iq_Filter2/1 -> Kiqcot2/1
  Kiqcot2/1 -> Ton_Sum2/2
  Ton_Sum2/1 -> Ton_Limit2/1
  Ton_Limit2/1 -> Ton_iqcot2/1
  IL_sample3/1 -> Abs3/1
  Abs3/1 -> ADC_Double3/1
  ADC_to_A3/1 -> Ierr3/2
  Ierr3/1 -> Iq_Filter3/1
  Iq_Filter3/1 -> Kiqcot3/1
  Kiqcot3/1 -> Ton_Sum3/2
  Ton_Sum3/1 -> Ton_Limit3/1
  Ton_Limit3/1 -> Ton_iqcot3/1
  IL_sample4/1 -> Abs4/1
  Abs4/1 -> ADC_Double4/1
  ADC_to_A4/1 -> Ierr4/2
  Ierr4/1 -> Iq_Filter4/1
  Iq_Filter4/1 -> Kiqcot4/1
  Kiqcot4/1 -> Ton_Sum4/2
  Ton_Sum4/1 -> Ton_Limit4/1
  Ton_Limit4/1 -> Ton_iqcot4/1
  ADC_Double1/1 -> ADC_to_A1/1
  ADC_Double2/1 -> ADC_to_A2/1
  ADC_Double3/1 -> ADC_to_A3/1
  ADC_Double4/1 -> ADC_to_A4/1
  Ton_trim1/1 -> Ton_Sum1/3
  Ton_trim2/1 -> Ton_Sum2/3
  Ton_trim3/1 -> Ton_Sum3/3
  Ton_trim4/1 -> Ton_Sum4/3
  Iref_Phase/1 -> Ierr1/1, Ierr2/1, Ierr3/1, Ierr4/1

== system four_phase_iek_dynamic_load_refslew/OnDelay ==
  u : Inport
  Compare To Constant : simulink/Logic and Bit Operations/Compare To Constant  relop=>=  const=Tdead  OutDataTypeStr=boolean
  Data Type Conversion : DataTypeConversion  OutDataTypeStr=double  SaturateOnIntegerOverflow=off  RndMeth=Floor
  Integrator : Integrator  ExternalReset=level
  Logical Operator : Logic  Operator=NOT  AllPortsSameDT=off  OutDataTypeStr=boolean
  y : Outport
  wires:
  u/1 -> Data Type Conversion/1, Logical Operator/1
  Logical Operator/1 -> Integrator/2
  Data Type Conversion/1 -> Integrator/1
  Integrator/1 -> Compare To Constant/1
  Compare To Constant/1 -> y/1

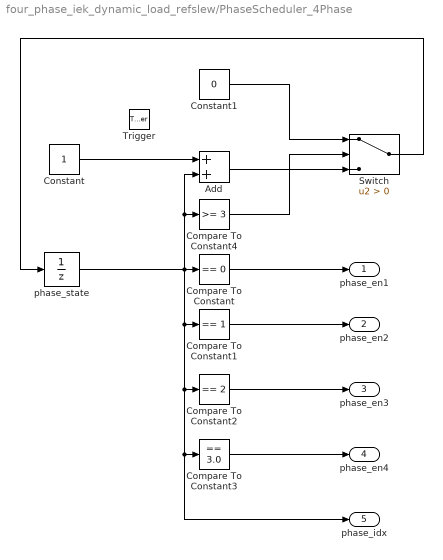
== system four_phase_iek_dynamic_load_refslew/PhaseScheduler_4Phase ==
  Trigger : TriggerPort  VariantControl=(inherit)
  Add : Sum
  Compare To Constant : simulink/Logic and Bit Operations/Compare To Constant  relop===  const=0  OutDataTypeStr=boolean
  Compare To Constant1 : simulink/Logic and Bit Operations/Compare To Constant  relop===  const=1  OutDataTypeStr=boolean
  Compare To Constant2 : simulink/Logic and Bit Operations/Compare To Constant  relop===  const=2  OutDataTypeStr=boolean
  Compare To Constant3 : simulink/Logic and Bit Operations/Compare To Constant  relop===  const=3.0  OutDataTypeStr=boolean
  Compare To Constant4 : simulink/Logic and Bit Operations/Compare To Constant  relop=>=  const=3  OutDataTypeStr=boolean
  Constant : Constant
  Constant1 : Constant  Value=0
  Switch : Switch  Criteria=u2 > Threshold  SaturateOnIntegerOverflow=off  InputSameDT=off
  phase_state : UnitDelay  SampleTime=-1  HasFrameUpgradeWarning=on
  phase_en1 : Outport
  phase_en2 : Outport  Port=2
  phase_en3 : Outport  Port=3
  phase_en4 : Outport  Port=4
  phase_idx : Outport  Port=5
  wires:
  phase_state/1 -> phase_idx/1, Compare To Constant3/1, Compare To Constant2/1, Compare To Constant1/1, Compare To Constant/1, Compare To Constant4/1, Add/2
  Compare To Constant/1 -> phase_en1/1
  Compare To Constant1/1 -> phase_en2/1
  Compare To Constant2/1 -> phase_en3/1
  Compare To Constant3/1 -> phase_en4/1
  Constant/1 -> Add/1
  Add/1 -> Switch/3
  Compare To Constant4/1 -> Switch/2
  Constant1/1 -> Switch/1
  Switch/1 -> phase_state/1

== system four_phase_iek_dynamic_load_refslew/GateDriver_1Phase1/OnDelay ==
  u : Inport
  Compare To Constant : simulink/Logic and Bit Operations/Compare To Constant  relop=>=  const=Tdead  OutDataTypeStr=boolean
  Data Type Conversion : DataTypeConversion  OutDataTypeStr=double  SaturateOnIntegerOverflow=off  RndMeth=Floor
  Integrator : Integrator  ExternalReset=level
  Logical Operator : Logic  Operator=NOT  AllPortsSameDT=off  OutDataTypeStr=boolean
  y : Outport
  wires:
  u/1 -> Data Type Conversion/1, Logical Operator/1
  Logical Operator/1 -> Integrator/2
  Data Type Conversion/1 -> Integrator/1
  Integrator/1 -> Compare To Constant/1
  Compare To Constant/1 -> y/1

== system four_phase_iek_dynamic_load_refslew/GateDriver_1Phase1/OnDelay1 ==
  u : Inport
  Compare To Constant : simulink/Logic and Bit Operations/Compare To Constant  relop=>=  const=Tdead  OutDataTypeStr=boolean
  Data Type Conversion : DataTypeConversion  OutDataTypeStr=double  SaturateOnIntegerOverflow=off  RndMeth=Floor
  Integrator : Integrator  ExternalReset=level
  Logical Operator : Logic  Operator=NOT  AllPortsSameDT=off  OutDataTypeStr=boolean
  y : Outport
  wires:
  u/1 -> Data Type Conversion/1, Logical Operator/1
  Logical Operator/1 -> Integrator/2
  Data Type Conversion/1 -> Integrator/1
  Integrator/1 -> Compare To Constant/1
  Compare To Constant/1 -> y/1

== system four_phase_iek_dynamic_load_refslew/GateDriver_1Phase2/OnDelay ==
  u : Inport
  Compare To Constant : simulink/Logic and Bit Operations/Compare To Constant  relop=>=  const=Tdead  OutDataTypeStr=boolean
  Data Type Conversion : DataTypeConversion  OutDataTypeStr=double  SaturateOnIntegerOverflow=off  RndMeth=Floor
  Integrator : Integrator  ExternalReset=level
  Logical Operator : Logic  Operator=NOT  AllPortsSameDT=off  OutDataTypeStr=boolean
  y : Outport
  wires:
  u/1 -> Data Type Conversion/1, Logical Operator/1
  Logical Operator/1 -> Integrator/2
  Data Type Conversion/1 -> Integrator/1
  Integrator/1 -> Compare To Constant/1
  Compare To Constant/1 -> y/1

== system four_phase_iek_dynamic_load_refslew/GateDriver_1Phase2/OnDelay1 ==
  u : Inport
  Compare To Constant : simulink/Logic and Bit Operations/Compare To Constant  relop=>=  const=Tdead  OutDataTypeStr=boolean
  Data Type Conversion : DataTypeConversion  OutDataTypeStr=double  SaturateOnIntegerOverflow=off  RndMeth=Floor
  Integrator : Integrator  ExternalReset=level
  Logical Operator : Logic  Operator=NOT  AllPortsSameDT=off  OutDataTypeStr=boolean
  y : Outport
  wires:
  u/1 -> Data Type Conversion/1, Logical Operator/1
  Logical Operator/1 -> Integrator/2
  Data Type Conversion/1 -> Integrator/1
  Integrator/1 -> Compare To Constant/1
  Compare To Constant/1 -> y/1

== system four_phase_iek_dynamic_load_refslew/GateDriver_1Phase3/OnDelay ==
  u : Inport
  Compare To Constant : simulink/Logic and Bit Operations/Compare To Constant  relop=>=  const=Tdead  OutDataTypeStr=boolean
  Data Type Conversion : DataTypeConversion  OutDataTypeStr=double  SaturateOnIntegerOverflow=off  RndMeth=Floor
  Integrator : Integrator  ExternalReset=level
  Logical Operator : Logic  Operator=NOT  AllPortsSameDT=off  OutDataTypeStr=boolean
  y : Outport
  wires:
  u/1 -> Data Type Conversion/1, Logical Operator/1
  Logical Operator/1 -> Integrator/2
  Data Type Conversion/1 -> Integrator/1
  Integrator/1 -> Compare To Constant/1
  Compare To Constant/1 -> y/1

== system four_phase_iek_dynamic_load_refslew/GateDriver_1Phase3/OnDelay1 ==
  u : Inport
  Compare To Constant : simulink/Logic and Bit Operations/Compare To Constant  relop=>=  const=Tdead  OutDataTypeStr=boolean
  Data Type Conversion : DataTypeConversion  OutDataTypeStr=double  SaturateOnIntegerOverflow=off  RndMeth=Floor
  Integrator : Integrator  ExternalReset=level
  Logical Operator : Logic  Operator=NOT  AllPortsSameDT=off  OutDataTypeStr=boolean
  y : Outport
  wires:
  u/1 -> Data Type Conversion/1, Logical Operator/1
  Logical Operator/1 -> Integrator/2
  Data Type Conversion/1 -> Integrator/1
  Integrator/1 -> Compare To Constant/1
  Compare To Constant/1 -> y/1

== system four_phase_iek_dynamic_load_refslew/GateDriver_1Phase4/OnDelay ==
  u : Inport
  Compare To Constant : simulink/Logic and Bit Operations/Compare To Constant  relop=>=  const=Tdead  OutDataTypeStr=boolean
  Data Type Conversion : DataTypeConversion  OutDataTypeStr=double  SaturateOnIntegerOverflow=off  RndMeth=Floor
  Integrator : Integrator  ExternalReset=level
  Logical Operator : Logic  Operator=NOT  AllPortsSameDT=off  OutDataTypeStr=boolean
  y : Outport
  wires:
  u/1 -> Data Type Conversion/1, Logical Operator/1
  Logical Operator/1 -> Integrator/2
  Data Type Conversion/1 -> Integrator/1
  Integrator/1 -> Compare To Constant/1
  Compare To Constant/1 -> y/1

== system four_phase_iek_dynamic_load_refslew/GateDriver_1Phase4/OnDelay1 ==
  u : Inport
  Compare To Constant : simulink/Logic and Bit Operations/Compare To Constant  relop=>=  const=Tdead  OutDataTypeStr=boolean
  Data Type Conversion : DataTypeConversion  OutDataTypeStr=double  SaturateOnIntegerOverflow=off  RndMeth=Floor
  Integrator : Integrator  ExternalReset=level
  Logical Operator : Logic  Operator=NOT  AllPortsSameDT=off  OutDataTypeStr=boolean
  y : Outport
  wires:
  u/1 -> Data Type Conversion/1, Logical Operator/1
  Logical Operator/1 -> Integrator/2
  Data Type Conversion/1 -> Integrator/1
  Integrator/1 -> Compare To Constant/1
  Compare To Constant/1 -> y/1
